simulink model "PTC_MBDS_DateTimeSource_Sample"  (R2013a)
settings: Solver=FixedStepDiscrete  SolverMode=SingleTasking  StartTime=0.0  StopTime=100  RelTol=1e-3  SampleTimeConstraint=Specified
libraries: PTC_MBDS_LIB x7, simulink_extras x1
settings Model: Creator=uidl7367  LastModifiedBy=Sundeep.Tuteja
settings DataIOCC: SignalLoggingSaveFormat=ModelDataLogs
settings OptimizationCC: ExpressionDepthLimit=2147483647  InitFltsAndDblsToZero=on
settings DebuggingCC: SaveWithParameterizedLinksMsg=none  SignalResolutionControl=TryResolveAllWithWarning  SolverPrmCheckMsg=none  InheritedTsInSrcMsg=none  MultiTaskDSMMsg=warning  MultiTaskCondExecSysMsg=none  FcnCallInpInsideContextMsg=UseLocalSettings  StrictBusMsg=Warning
settings RTWCC: IncludeERTFirstTime=on
settings GRTTargetCC: TargetFcnLib=ansi_tfl_tmw.mat  CombineOutputUpdateFcns=off  GRTInterface=on

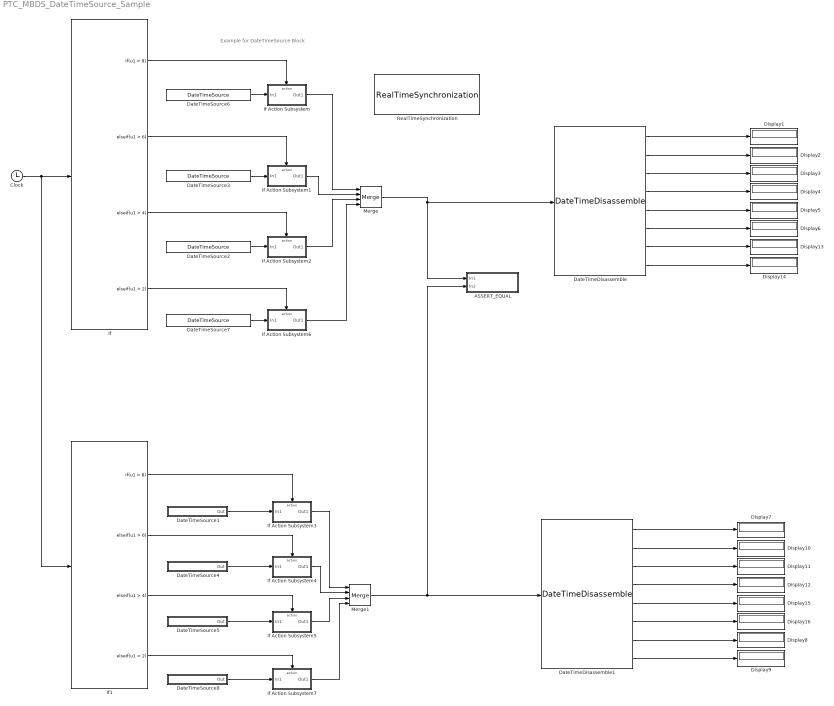
== system PTC_MBDS_DateTimeSource_Sample ==
  note: Example for DateTimeSource Block
  ASSERT_EQUAL : Subsystem
  Clock : Clock
  DateTimeDisassemble : PTC_MBDS_LIB/MBDS Standard Library/Extended Operations/Date & Time Operations/Date & Time Conversions/DateTimeDisassemble  ENO_Enabled=on  PTC_MBDS_BlockVersion=5.40  PTC_BlockType=PTC_MBDS_DateTimeDisassemble
  DateTimeDisassemble1 : PTC_MBDS_LIB/MBDS Standard Library/Extended Operations/Date & Time Operations/Date & Time Conversions/DateTimeDisassemble  ENO_Enabled=on  PTC_MBDS_BlockVersion=5.40  PTC_BlockType=PTC_MBDS_DateTimeDisassemble
  DateTimeSource1 : Subsystem  InitFcn=|  mask(DateTimeSource){MBDS_LibraryBlock=on, InputValue=1986-11-10-11:05:04, MBDS_BlockVersion=05.40}
      | if(exist('MBDS_BlockCallback', 'file'))
      |    MBDS_BlockCallback('Update', gcb);
      | end
      mask prompts: MBDS_LibraryBlock "MBDS Library Block"; InputValue "Constant value:"; MBDS_BlockVersion "Block version:"
      mask help: This block outputs a constant date and time signal based on a uint32 data type. Specify the date and time by the 'Constant value' parameter. Comply to the format: 2000-12-24-20:01:23.
      mask init:
      | MBDS_BlockCallback('Copy', gcb);
      | Text = InputValue;
      | try
      |    % Try to evaluate project constant 
      |    EvalValue = evalin('base', InputValue);
      |    if(~isempty(EvalValue))
      |       InputValue = EvalValue;
      |    end
      | end
      | % Convert string to value (enable silent mode)
      | Value = ConvertSignalValue(InputValue, 'date_time', 'Str2Val', true);
      mask Help: eval(['open([workdir(''Library_Dir:''),''\Blockset\Help\'',get_param(gcb,''MaskType''),''.html''])'])
      mask Display: disp([' ',Text,' ']);
  DateTimeSource2 : PTC_MBDS_LIB/MBDS Standard Library/Extended Operations/Date & Time Operations/DateTimeSource  InputValue=2007-07-14-11:05:04  PTC_MBDS_BlockVersion=5.40  PTC_BlockType=PTC_MBDS_DateTimeSource  Value=1184411104
  DateTimeSource3 : PTC_MBDS_LIB/MBDS Standard Library/Extended Operations/Date & Time Operations/DateTimeSource  InputValue=2007-07-13-11:05:04  PTC_MBDS_BlockVersion=5.40  PTC_BlockType=PTC_MBDS_DateTimeSource  Value=1184324704
  DateTimeSource4 : Subsystem  InitFcn=|  mask(DateTimeSource){MBDS_LibraryBlock=on, InputValue=2007-07-13-11:05:04, MBDS_BlockVersion=05.40}
      | if(exist('MBDS_BlockCallback', 'file'))
      |    MBDS_BlockCallback('Update', gcb);
      | end
      mask prompts: MBDS_LibraryBlock "MBDS Library Block"; InputValue "Constant value:"; MBDS_BlockVersion "Block version:"
      mask help: This block outputs a constant date and time signal based on a uint32 data type. Specify the date and time by the 'Constant value' parameter. Comply to the format: 2000-12-24-20:01:23.
      mask init: same as PTC_MBDS_DateTimeSource_Sample/DateTimeSource1
      mask Help: eval(['open([workdir(''Library_Dir:''),''\Blockset\Help\'',get_param(gcb,''MaskType''),''.html''])'])
      mask Display: disp([' ',Text,' ']);
  DateTimeSource5 : Subsystem  InitFcn=|  mask(DateTimeSource){MBDS_LibraryBlock=on, InputValue=2007-07-14-11:05:04, MBDS_BlockVersion=05.40}
      | if(exist('MBDS_BlockCallback', 'file'))
      |    MBDS_BlockCallback('Update', gcb);
      | end
      mask prompts: MBDS_LibraryBlock "MBDS Library Block"; InputValue "Constant value:"; MBDS_BlockVersion "Block version:"
      mask help: This block outputs a constant date and time signal based on a uint32 data type. Specify the date and time by the 'Constant value' parameter. Comply to the format: 2000-12-24-20:01:23.
      mask init: same as PTC_MBDS_DateTimeSource_Sample/DateTimeSource1
      mask Help: eval(['open([workdir(''Library_Dir:''),''\Blockset\Help\'',get_param(gcb,''MaskType''),''.html''])'])
      mask Display: disp([' ',Text,' ']);
  DateTimeSource6 : PTC_MBDS_LIB/MBDS Standard Library/Extended Operations/Date & Time Operations/DateTimeSource  InputValue=1986-11-10-11:05:04  PTC_MBDS_BlockVersion=5.40  PTC_BlockType=PTC_MBDS_DateTimeSource  Value=532004704
  DateTimeSource7 : PTC_MBDS_LIB/MBDS Standard Library/Extended Operations/Date & Time Operations/DateTimeSource  InputValue=2007-12-01-11:05:04  PTC_MBDS_BlockVersion=5.40  PTC_BlockType=PTC_MBDS_DateTimeSource  Value=1196507104
  DateTimeSource8 : Subsystem  InitFcn=|  mask(DateTimeSource){MBDS_LibraryBlock=on, InputValue=2007-11-31-11:05:04, MBDS_BlockVersion=05.40}
      | if(exist('MBDS_BlockCallback', 'file'))
      |    MBDS_BlockCallback('Update', gcb);
      | end
      mask prompts: MBDS_LibraryBlock "MBDS Library Block"; InputValue "Constant value:"; MBDS_BlockVersion "Block version:"
      mask help: This block outputs a constant date and time signal based on a uint32 data type. Specify the date and time by the 'Constant value' parameter. Comply to the format: 2000-12-24-20:01:23.
      mask init: same as PTC_MBDS_DateTimeSource_Sample/DateTimeSource1
      mask Help: eval(['open([workdir(''Library_Dir:''),''\Blockset\Help\'',get_param(gcb,''MaskType''),''.html''])'])
      mask Display: disp([' ',Text,' ']);
  Display{1..16} (16 alike) : Display
  If : If  IfExpression=u1 > 8  ElseIfExpressions=u1 > 6, u1 > 4, u1 > 2  ShowElse=off
  If Action Subsystem : Subsystem  TreatAsAtomicUnit=on
  If Action Subsystem1 : Subsystem  TreatAsAtomicUnit=on
  If Action Subsystem2 : Subsystem  TreatAsAtomicUnit=on
  If Action Subsystem3 : Subsystem  TreatAsAtomicUnit=on
  If Action Subsystem4 : Subsystem  TreatAsAtomicUnit=on
  If Action Subsystem5 : Subsystem  TreatAsAtomicUnit=on
  If Action Subsystem6 : Subsystem  TreatAsAtomicUnit=on
  If Action Subsystem7 : Subsystem  TreatAsAtomicUnit=on
  If1 : If  IfExpression=u1 > 8  ElseIfExpressions=u1 > 6, u1 > 4, u1 > 2  ShowElse=off
  Merge : Merge  Inputs=4
  Merge1 : Merge  Inputs=4
  RealTimeSynchronization : PTC_MBDS_LIB/MBDS Standard Library/Extended Operations/HMI/RealTimeSynchronization  Enable=off  PTC_MBDS_BlockVersion=5.40  PTC_BlockType=PTC_MBDS_RealTimeSynchronization
  wires:
  Clock/1 -> If1/1, If/1
  If/1 -> If Action Subsystem/Action
  DateTimeSource6/1 -> If Action Subsystem/1(In1)
  DateTimeSource3/1 -> If Action Subsystem1/1(In1)
  DateTimeSource2/1 -> If Action Subsystem2/1(In1)
  If Action Subsystem1/1(Out1) -> Merge/2
  If Action Subsystem2/1(Out1) -> Merge/3
  If Action Subsystem/1(Out1) -> Merge/1
  Merge/1 -> ASSERT_EQUAL/1(In1), DateTimeDisassemble/1
  If/2 -> If Action Subsystem1/Action
  If/3 -> If Action Subsystem2/Action
  DateTimeSource1/1(Out) -> If Action Subsystem3/1(In1)
  DateTimeSource4/1(Out) -> If Action Subsystem4/1(In1)
  DateTimeSource5/1(Out) -> If Action Subsystem5/1(In1)
  If Action Subsystem4/1(Out1) -> Merge1/2
  If Action Subsystem5/1(Out1) -> Merge1/3
  If Action Subsystem3/1(Out1) -> Merge1/1
  Merge1/1 -> DateTimeDisassemble1/1, ASSERT_EQUAL/2(In2)
  If1/1 -> If Action Subsystem3/Action
  If1/2 -> If Action Subsystem4/Action
  If1/3 -> If Action Subsystem5/Action
  If/4 -> If Action Subsystem6/Action
  DateTimeSource7/1 -> If Action Subsystem6/1(In1)
  If1/4 -> If Action Subsystem7/Action
  DateTimeSource8/1(Out) -> If Action Subsystem7/1(In1)
  If Action Subsystem6/1(Out1) -> Merge/4
  If Action Subsystem7/1(Out1) -> Merge1/4
  DateTimeDisassemble/8 -> Display14/1
  DateTimeDisassemble/1 -> Display1/1
  DateTimeDisassemble/3 -> Display3/1
  DateTimeDisassemble/2 -> Display2/1
  DateTimeDisassemble/4 -> Display4/1
  DateTimeDisassemble/6 -> Display6/1
  DateTimeDisassemble/5 -> Display5/1
  DateTimeDisassemble/7 -> Display13/1
  DateTimeDisassemble1/8 -> Display9/1
  DateTimeDisassemble1/1 -> Display7/1
  DateTimeDisassemble1/3 -> Display11/1
  DateTimeDisassemble1/2 -> Display10/1
  DateTimeDisassemble1/4 -> Display12/1
  DateTimeDisassemble1/6 -> Display16/1
  DateTimeDisassemble1/5 -> Display15/1
  DateTimeDisassemble1/7 -> Display8/1

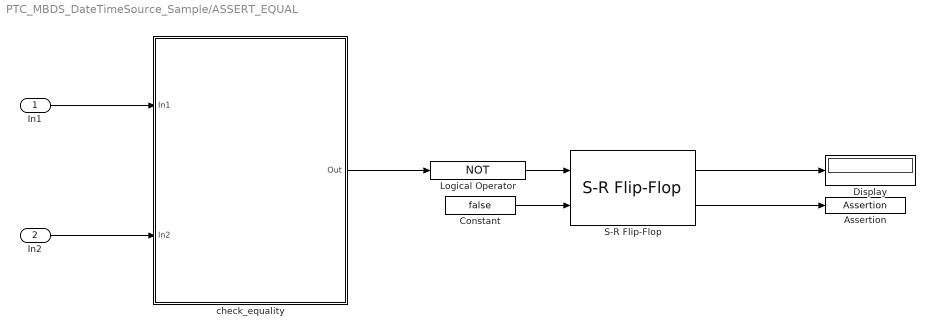
== system PTC_MBDS_DateTimeSource_Sample/ASSERT_EQUAL ==
  In1 : Inport
  In2 : Inport  Port=2
  Assertion : Assertion
  Constant : Constant  Value=false
  Display : Display
  Logical Operator : Logic  Operator=NOT  AllPortsSameDT=off  OutDataTypeStr=boolean
  S-R Flip-Flop : simulink_extras/Flip Flops/S-R Flip-Flop  initial_condition=0
  check_equality : MATLAB Function  TreatAsAtomicUnit=on
  wires:
  S-R Flip-Flop/1 -> Display/1
  check_equality/1(Out) -> Logical Operator/1
  Constant/1 -> S-R Flip-Flop/2
  S-R Flip-Flop/2 -> Assertion/1
  In2/1 -> check_equality/2(In2)
  In1/1 -> check_equality/1(In1)
  Logical Operator/1 -> S-R Flip-Flop/1

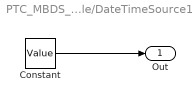
== system PTC_MBDS_DateTimeSource_Sample/DateTimeSource1 ==
  Constant : Constant  Value=Value  OutDataTypeStr=uint32  LockScale=on
  Out : Outport
  wires:
  Constant/1 -> Out/1

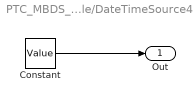
== system PTC_MBDS_DateTimeSource_Sample/DateTimeSource4 ==
  Constant : Constant  Value=Value  OutDataTypeStr=uint32  LockScale=on
  Out : Outport
  wires:
  Constant/1 -> Out/1

== system PTC_MBDS_DateTimeSource_Sample/DateTimeSource5 ==
  Constant : Constant  Value=Value  OutDataTypeStr=uint32  LockScale=on
  Out : Outport
  wires:
  Constant/1 -> Out/1

== system PTC_MBDS_DateTimeSource_Sample/DateTimeSource8 ==
  Constant : Constant  Value=Value  OutDataTypeStr=uint32  LockScale=on
  Out : Outport
  wires:
  Constant/1 -> Out/1

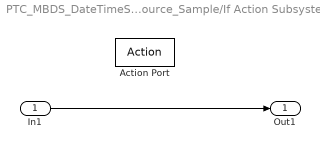
== system PTC_MBDS_DateTimeSource_Sample/If Action Subsystem ==
  In1 : Inport
  Action Port : ActionPort  ActionType=then
  Out1 : Outport
  wires:
  In1/1 -> Out1/1

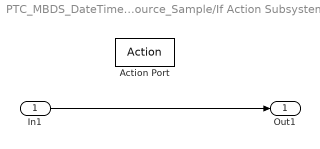
== system PTC_MBDS_DateTimeSource_Sample/If Action Subsystem1 ==
  In1 : Inport
  Action Port : ActionPort  ActionType=elseif
  Out1 : Outport
  wires:
  In1/1 -> Out1/1

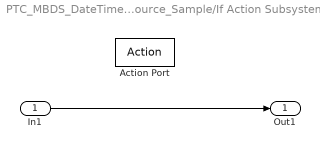
== system PTC_MBDS_DateTimeSource_Sample/If Action Subsystem2 ==
  In1 : Inport
  Action Port : ActionPort  ActionType=elseif
  Out1 : Outport
  wires:
  In1/1 -> Out1/1

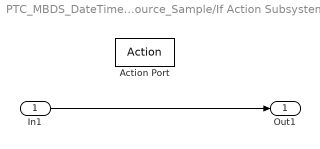
== system PTC_MBDS_DateTimeSource_Sample/If Action Subsystem3 ==
  In1 : Inport
  Action Port : ActionPort  ActionType=then
  Out1 : Outport
  wires:
  In1/1 -> Out1/1

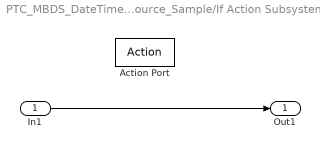
== system PTC_MBDS_DateTimeSource_Sample/If Action Subsystem4 ==
  In1 : Inport
  Action Port : ActionPort  ActionType=elseif
  Out1 : Outport
  wires:
  In1/1 -> Out1/1

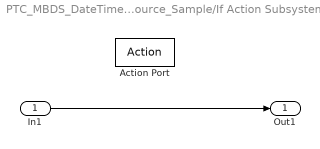
== system PTC_MBDS_DateTimeSource_Sample/If Action Subsystem5 ==
  In1 : Inport
  Action Port : ActionPort  ActionType=elseif
  Out1 : Outport
  wires:
  In1/1 -> Out1/1

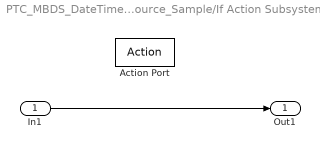
== system PTC_MBDS_DateTimeSource_Sample/If Action Subsystem6 ==
  In1 : Inport
  Action Port : ActionPort  ActionType=elseif
  Out1 : Outport
  wires:
  In1/1 -> Out1/1

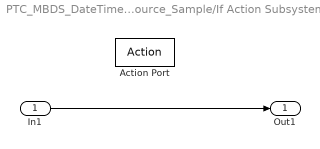
== system PTC_MBDS_DateTimeSource_Sample/If Action Subsystem7 ==
  In1 : Inport
  Action Port : ActionPort  ActionType=elseif
  Out1 : Outport
  wires:
  In1/1 -> Out1/1

== matlab function PTC_MBDS_DateTimeSource_Sample/ASSERT_EQUAL/check_equality ==
  data: In1 input; Out output; In2 input
function Out = check_equality(In1, In2)
%#codegen

Out = isequaln(In1, In2);

end
